simulink model "bell_nexus_4ex_model_ol"  (R2024a)
settings: Solver=ode4  StartTime=0.0  StopTime=simt  FixedStep=st  RelTol=1e-3
model workspace (MAT data in the model file):
  aaaa = [0 0 0 0]
  init_lat = [0 0 0 1]
values from neighbouring files (symbols this model uses):
  B_lat_ext = [B_lat, Bw_lat]    [bell_nexus_4ex.m]
  B_lon_ext = [B_lon, Bw_lon]    [bell_nexus_4ex.m]
  C_lat_ext = [C_lat; eye(1,4)]    [bell_nexus_4ex.m]
  C_lon_ext = [C_lon; eye(2,4)]    [bell_nexus_4ex.m]
  D_lat_ext = blkdiag(D_lat, Tw_lat(1,:))    [bell_nexus_4ex.m]
  D_lon_ext = blkdiag(D_lon, Tw_lon(1:2,:))    [bell_nexus_4ex.m]
  w_st_time = 4    [bell_nexus_4ex.m]
  wind_lat = [0 0 0]    [bell_nexus_4ex.m]
  wind_lon = [0 0 0]    [bell_nexus_4ex.m]
undefined symbols (not defined in the file or in its folder): A_lat, A_lon
settings Model: Creator=pries  LastModifiedBy=pries
settings RTWCC: GPUComputeCapability=3.5

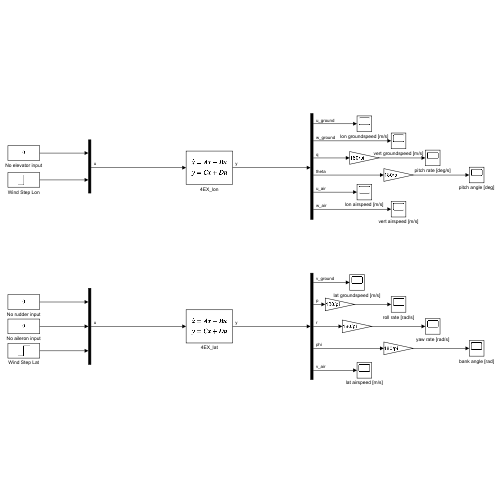
[thumbnail: Simulink's stored preview of the top-level diagram]
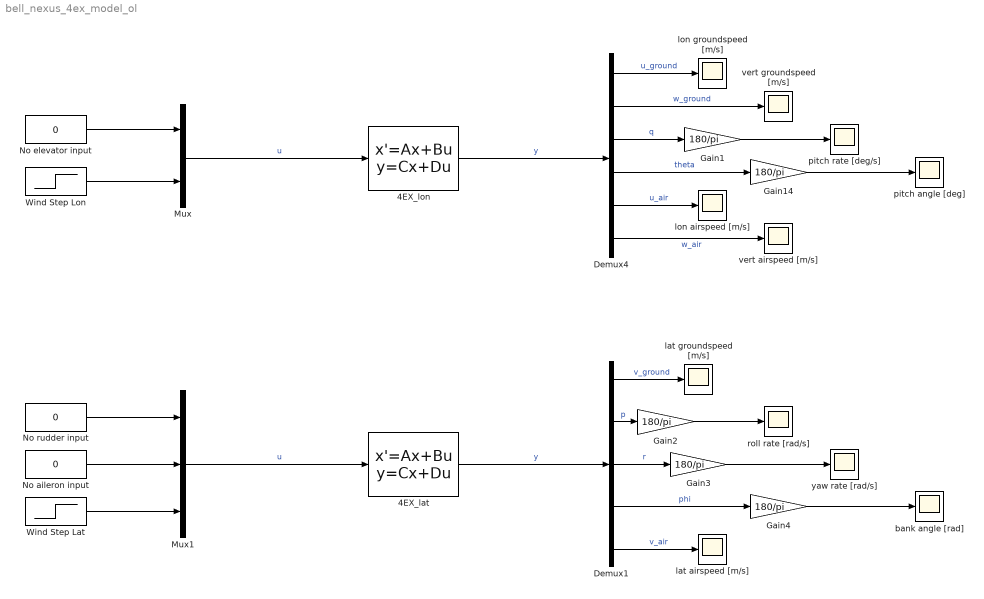
== system bell_nexus_4ex_model_ol ==
  4EX_lat : StateSpace  A=A_lat  B=B_lat_ext  C=C_lat_ext  D=D_lat_ext  InitialCondition=[0 0 0 0]  ParameterTunability=Unconstrained
  4EX_lon : StateSpace  A=A_lon  B=B_lon_ext  C=C_lon_ext  D=D_lon_ext  InitialCondition=[0 0 0 0]  ParameterTunability=Unconstrained
  Demux1 : Demux  Outputs=5
  Demux4 : Demux  Outputs=6
  Gain{1..4,14} (5 alike) : Gain  Gain=180/pi
  Mux : Mux  Inputs=2
  Mux1 : Mux  Inputs=3
  No aileron input : Constant  Value=0
  No elevator input : Constant  Value=0
  No rudder input : Constant  Value=0
  Wind Step Lat : Step  Time=w_st_time  Before=[0 0 0]  After=wind_lat  SampleTime=0
  Wind Step Lon : Step  Time=w_st_time  Before=[0 0 0]  After=wind_lon  SampleTime=0
  bank angle [rad] : Scope
  lat airspeed [m/s] : Scope
  lat groundspeed [m/s] : Scope
  lon airspeed [m/s] : Scope
  lon groundspeed [m/s] : Scope
  pitch angle [deg] : Scope
  pitch rate [deg/s] : Scope
  roll rate [rad/s] : Scope
  vert airspeed [m/s] : Scope
  vert groundspeed [m/s] : Scope
  yaw rate [rad/s] : Scope
  wires:
  Demux4/4 -> Gain14/1  "theta"
  4EX_lon/1 -> Demux4/1  "y"
  Demux4/2 -> vert groundspeed [m/s]/1  "w_ground"
  Demux4/3 -> Gain1/1  "q"
  Demux4/1 -> lon groundspeed [m/s]/1  "u_ground"
  Demux4/5 -> lon airspeed [m/s]/1  "u_air"
  Demux4/6 -> vert airspeed [m/s]/1  "w_air"
  Mux/1 -> 4EX_lon/1  "u"
  No elevator input/1 -> Mux/1
  Demux1/1 -> lat groundspeed [m/s]/1  "v_ground"
  Demux1/5 -> lat airspeed [m/s]/1  "v_air"
  Demux1/4 -> Gain4/1  "phi"
  Demux1/2 -> Gain2/1  "p"
  Demux1/3 -> Gain3/1  "r"
  4EX_lat/1 -> Demux1/1  "y"
  Wind Step Lon/1 -> Mux/2
  Mux1/1 -> 4EX_lat/1  "u"
  Wind Step Lat/1 -> Mux1/3
  No aileron input/1 -> Mux1/2
  No rudder input/1 -> Mux1/1
  Gain14/1 -> pitch angle [deg]/1
  Gain1/1 -> pitch rate [deg/s]/1
  Gain2/1 -> roll rate [rad/s]/1
  Gain3/1 -> yaw rate [rad/s]/1
  Gain4/1 -> bank angle [rad]/1
